simulink model "simulink_TP_3"  (R2017b)
settings: Solver=VariableStepAuto  StartTime=0.0  StopTime=10.0  RelTol=1e-3
InitFcn:
  | constantes3
values from neighbouring files (symbols this model uses):
  J = 3.2284*10^(-6)    (= 3.2284e-06)    [constantes.m]    (also in constantes2.m = 0.28; constantes3.m = 0.2; constantes_ABS.m = 0.5)
  L = 2.75*10^(-6)    (= 2.75e-06)    [constantes.m]    (also in constantes2.m = 0.0016; constantes3.m = 9.161)
  P = 3    [constantes3.m]
undefined symbols (not defined in the file or in its folder): Phi
settings Model: Creator=Table2  LastModifiedBy=Table2

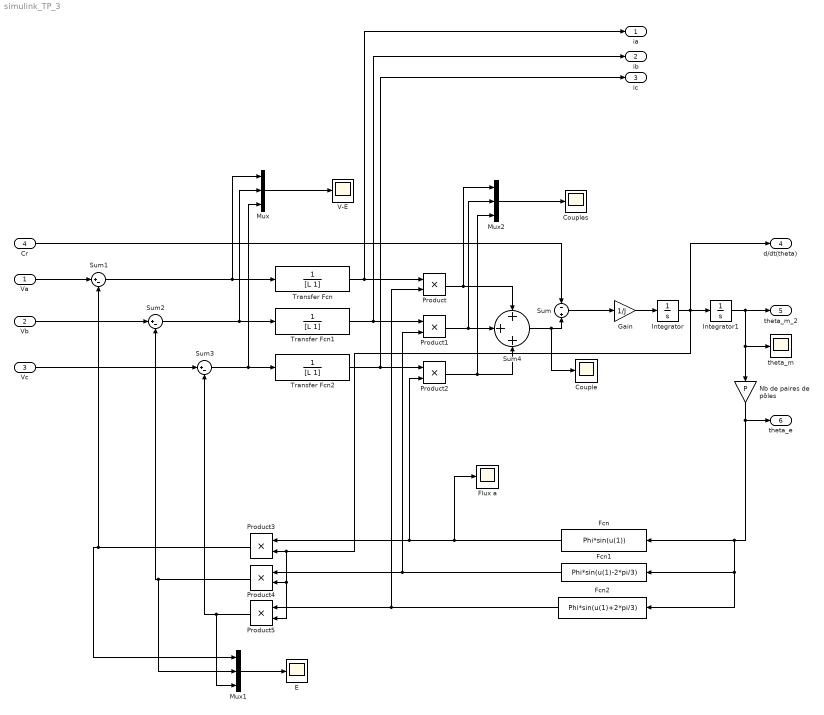
== system simulink_TP_3 ==
  Va : Inport
  Vb : Inport  Port=2
  Vc : Inport  Port=3
  Cr : Inport  Port=4
  Couple : Scope
  Couples : Scope
  E : Scope
  Fcn : Fcn  Expr=Phi*sin(u(1))
  Fcn1 : Fcn  Expr=Phi*sin(u(1)-2*pi/3)
  Fcn2 : Fcn  Expr=Phi*sin(u(1)+2*pi/3)
  Flux a : Scope
  Gain : Gain  Gain=1/J
  Integrator : Integrator
  Integrator1 : Integrator
  Mux : Mux  Inputs=3
  Mux1 : Mux  Inputs=3
  Mux2 : Mux  Inputs=3
  Nb de paires de pôles : Gain  Gain=P
  Product{,1..5} (6 alike) : Product
  Sum : Sum  Inputs=-|+
  Sum1 : Sum  Inputs=|+-
  Sum2 : Sum  Inputs=|+-
  Sum3 : Sum  Inputs=|+-
  Sum4 : Sum  Inputs=+++
  Transfer Fcn : TransferFcn  Denominator=[L 1]
  Transfer Fcn1 : TransferFcn  Denominator=[L 1]
  Transfer Fcn2 : TransferFcn  Denominator=[L 1]
  V-E : Scope
  theta_m : Scope
  ia : Outport
  ib : Outport  Port=2
  ic : Outport  Port=3
  d/dt(theta) : Outport  Port=4
  theta_m_2 : Outport  Port=5
  theta_e : Outport  Port=6
  wires:
  Va/1 -> Sum1/1
  Vb/1 -> Sum2/1
  Vc/1 -> Sum3/1
  Sum1/1 -> Mux/1, Transfer Fcn/1
  Sum2/1 -> Mux/2, Transfer Fcn1/1
  Sum3/1 -> Mux/3, Transfer Fcn2/1
  Mux/1 -> V-E/1
  Sum4/1 -> Couple/1, Sum/2
  Product1/1 -> Mux2/2, Sum4/2
  Product/1 -> Mux2/1, Sum4/1
  Product2/1 -> Mux2/3, Sum4/3
  Transfer Fcn2/1 -> ic/1, Product2/1
  Transfer Fcn1/1 -> ib/1, Product1/1
  Transfer Fcn/1 -> ia/1, Product/1
  Mux2/1 -> Couples/1
  Cr/1 -> Sum/1
  Sum/1 -> Gain/1
  Gain/1 -> Integrator/1
  Integrator1/1 -> theta_m/1, Nb de paires de pôles/1, theta_m_2/1
  Nb de paires de pôles/1 -> theta_e/1, Fcn2/1, Fcn1/1, Fcn/1
  Fcn/1 -> Flux a/1, Product2/2, Product3/1
  Fcn1/1 -> Product1/2, Product4/1
  Fcn2/1 -> Product/2, Product5/1
  Integrator/1 -> d/dt(theta)/1, Product5/2, Product4/2, Product3/2, Integrator1/1
  Mux1/1 -> E/1
  Product3/1 -> Mux1/1, Sum1/2
  Product4/1 -> Mux1/2, Sum2/2
  Product5/1 -> Mux1/3, Sum3/2
